simulink model "MicroMouseTemplate"  (R2024b)
settings: Solver=FixedStepAuto  StartTime=0.0  StopTime=10.0  RelTol=1e-3  EnableMultiTasking=on
undefined symbols (not defined in the file): samplingTime
settings Model: STM32="{\"DigitalPortRead\":[{\"ID\":\"MicroMouseTemplate:2483:4\"},{\"ID\":\"MicroMouseTemplate:2483:3\"}],\"DigitalPortWrite\":[{\"ID\":\"MicroMouseTemplate:84:10\"},{\"ID\":\"MicroMouseTemplate:84:9\"},{\"ID\":\"MicroMouseTemplate:84:8\"},{\"ID\":\"MicroMouseTemplate:84:7\"},{\"ID\":\"MicroMouseTemplate:84:6\"},{\"ID\":\"MicroMouseTemplate:84:5\"},{\"ID\":\"MicroMouseTemplate:84:4\"},{\"ID\":\"MicroMouseTemplate:84:3\"},{\"ID\":\"MicroMouseTemplate:2479:8\"},{\"ID\":\"MicroMouseTemplate:2479:7\"},{\"ID\":\"MicroMouseTemplate:2479:6\"},{\"ID\":\"MicroMouseTemplate:2479:4\"},{\"ID\":\"MicroMouseTemplate:160:19\"}],\"PWMOutput\":[{\"ID\":\"MicroMouseTemplate:160:25\"},{\"ID\":\"MicroMouseTemplate:160:24\"}],\"AnalogInput\":{\"ID\":\"MicroMouseTemplate:2357:1\"}}"  SimulationMode=external  ExtModeTrigDuration=10  Creator=JesseJabezArendse  LastModifiedBy=emanu
settings SolverCC: AllowMultiTaskInputOutput=on  AutoInsertRateTranBlk=on  InsertRTBMode=Never (minimum delay)
settings OptimizationCC: EnhancedBackFolding=on  PassReuseOutputArgsAs=Individual arguments  StateBitsets=on  DataBitsets=on  ZeroExternalMemoryAtStartup=off  ZeroInternalMemoryAtStartup=off  NoFixptDivByZeroProtection=on  MaxStackSize=512  OptimizeBlockOrder=speed  DifferentSizesBufferReuse=on  EfficientTunableParamExpr=on
settings DebuggingCC: MultiTaskCondExecSysMsg=none  ParameterOverflowMsg=none  ParameterPrecisionLossMsg=none  ParameterTunabilityLossMsg=error
settings HardwareCC: ProdBitPerPointer=32  ProdBitPerSizeT=32  ProdBitPerPtrDiffT=32  ProdLargestAtomicInteger=Long  ProdLargestAtomicFloat=Double  ProdWordSize=32  ProdLongLongMode=on  ProdHWDeviceType=ARM Compatible->ARM Cortex  TargetBitPerPointer=64  TargetBitPerSizeT=64  TargetBitPerPtrDiffT=64  TargetLongLongMode=on  TargetIntDivRoundTo=Zero  TargetEndianess=LittleEndian  TargetWordSize=64  TargetHWDeviceType=MATLAB Host
settings ModelReferenceCC: EnableParallelModelReferenceBuilds=on  ParallelModelReferenceMATLABWorkerInit=Copy Base Workspace  SupportModelReferenceSimTargetCustomCode=on
settings SFSimCC: MATLABDynamicMemAlloc=off  SimHardwareAcceleration=native
settings RTWCC: Description=Embedded Coder  SystemTargetFile=ert.tlc  HardwareBoard=STM32L4xx Based  TLCOptions=-p0 -aInlineSetEventsForThisBaseRateFcn=TLC_FALSE -aSuppressMultiTaskScheduler=TLC_FALSE -aRateBasedStepFcn=1  TemplateMakefile=ert_default_tmf  Toolchain=GNU Tools for ARM Embedded Processors  CodeExecutionProfiling=on  CodeProfilingInstrumentation=coarse  GPUComputeCapability=3.5
settings RTWCC: CustomHeaderCode=|
  | #include "MicroMouseProgramming\Core\Inc\IMU.h"
  | #include "MicroMouseProgramming\Core\Inc\CustomWhile.h"
  | #include "MicroMouseProgramming\Core\Inc\Motors.h"
settings RTWCC: CustomInclude=|
  | MicroMouseProgramming\Core\Inc\
  | MicroMouseProgramming\Core\Src\
settings RTWCC: CustomSource=|
  | MicroMouseProgramming\Core\Src\IMU.c
  | MicroMouseProgramming\Core\Src\CustomWhile.c
  | MicroMouseProgramming\Core\Src\Motors.c
settings CodeAppCC: ForceParamTrailComments=on  IgnoreCustomStorageClasses=off  OperatorAnnotations=on  SimulinkDataObjDesc=on  SFDataObjDesc=on  InsertBlockDesc=on
settings ERTTargetCC: CodeReplacementLibrary=ARM Cortex-M  SupportNonFinite=off  SupportComplex=off  ExtModeTransport=3  ExtModeStaticAlloc=on  ExtModeStaticAllocSize=2048  ExtModeMexFile=ext_xcp  ExtModeIntrfLevel=Level2 - Open  InlinedParameterPlacement=Hierarchical  DynamicArrayContainerType=coder::array

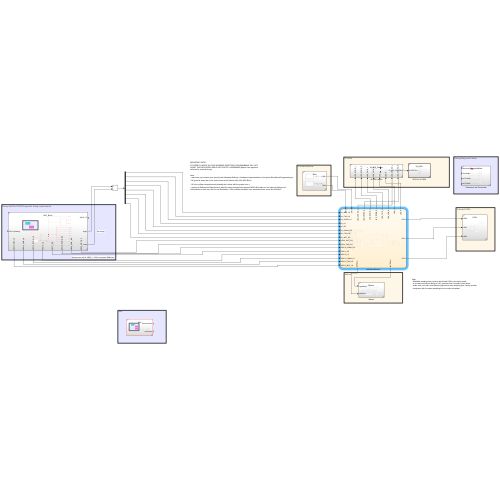
[thumbnail: Simulink's stored preview of the top-level diagram]
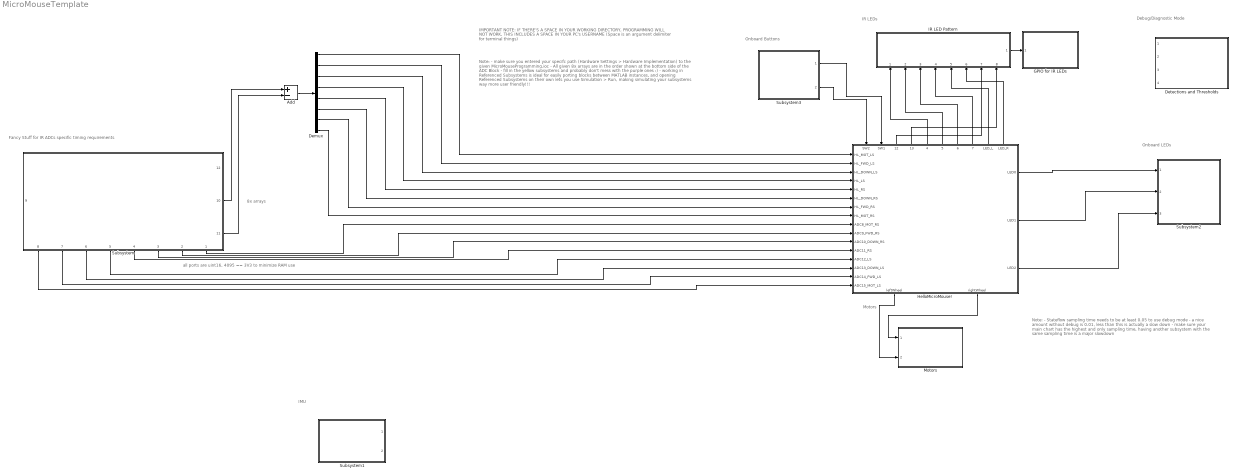
== system MicroMouseTemplate ==
  note: IMPORTANT NOTE:
      | IF THERE'S A SPACE IN YOUR WORKING DIRECTORY, PROGRAMMING WILL NOT WORK, THIS INCLUDES A SPACE IN YOUR PC's USERNAME (Space is an argument delimiter for terminal things)
  note: Note:
      | - make sure you entered your specifc path (Hardware Settings > Hardware Implementation) to the given MicroMouseProgramming.ioc
      | - All given 8x arrays are in the order shown at the bottom side of the ADC Block
      |
      | - fill in the yellow subsystems and probably don't mess with the purple ones :)
      | - working in Referenced Subsystems is ideal for easily porting blocks between MATLAB instances, and opening Referenced Subsystems on their own lets you use Simulation > Run, making simulating your subsystems way more user friendly!!!
  note: 8x arrays
  note: all ports are uint16, 4095 == 3V3 to minimize RAM use
  note: IMU
  note: Note:
      | - Stateflow sampling time needs to be at least 0.05 to use debug mode
      | - a nice amount without debug is 0.01, less than this is actually a slow down
      | - make sure your main chart has the highest and only sampling time, having another
      | subsystem with the same sampling time is a major slowdown
  note: Fancy Stuff for IR ADCs specific timing requirements
  note: IR LEDs
  note: Motors
  note: Onboard Buttons
  note: Onboard LEDs
  note: Debug/Diagnostic Mode
  Add : Sum  Inputs=+-
  Demux : Demux  Outputs=8
  Detections and Thresholds : Subsystem  ReferencedSubsystem=DiagnosticMode
  GPIO for IR LEDs : Subsystem  TreatAsAtomicUnit=on  SystemSampleTime=samplingTime  ReferencedSubsystem=IR_LEDs
  HelloMicroMouse! : Stateflow chart  TreatAsAtomicUnit=on
      settings: PortSchema="{\"entries\":[{\"content\":{\"sides\":[{\"content\":{\"connectorIds\":[\"In1\",\"In2\",\"In3\",\"In4\",\"In5\",\"In6\",\"In7\",\"In8\",\"In9\",\"In14\",\"In18\",\"In13\",\"In12\",\"In17\",\"In11\",\"In10\"]},\"type\":\"ConnectorPlacement.EquallySpacedRectSide\",\"uuid\":\"f52daa4f-6374-42e5-9ef1-0ccc99d09b58\"},{\"content\":{\"connectorIds\":[\"Out1\",\"Out10\",\"Out11\"],\"side\":\"RIGHT\"},\"type\":\"ConnectorPlacement.EquallySpacedRectSide\",\"uuid\":\"94b478cc-4dde-45c7-a588-77cf2b43cdb7\"},{\"content\":{\"connectorIds\":[\"In15\",\"In16\",\"Out12\",\"Out13\",\"Out4\",\"Out5\",\"Out6\",\"Out7\",\"Out8\",\"Out9\"],\"side\":\"TOP\"},\"type\":\"ConnectorPlacement.EquallySpacedRectSide\",\"uuid\":\"afff2079-ea5c-423e-9722-09c3bbce433b\"},{\"content\":{\"connectorIds\":[\"Out2\",\"Out3\"],\"side\":\"BOTTOM\"},\"type\":\"ConnectorPlacement.EquallySpacedRectSide\",\"uuid\":\"94e93a1d-795d-41a3-b2d8-d520b2bf47ef\"}]},\"type\":\"ConnectorPlacement.EquallySpacedConnector\",\"uuid\":\"d4d35636-54af-48ac-af70-d56caef5e090\"}],\"packageUris\":[\"http://schema.mathworks.com/mf0/Connector/R2020b\"],\"version\":\"1.0\"}"
  IR LED Pattern : Subsystem  ReferencedSubsystem=IR_LED_Pattern
      settings: PortSchema="{\"entries\":[{\"content\":{\"sides\":[{\"content\":{},\"type\":\"ConnectorPlacement.EquallySpacedRectSide\",\"uuid\":\"bebb72a7-933c-42e2-8276-ac4f31a32b24\"},{\"content\":{\"connectorIds\":[\"Out1\"],\"side\":\"RIGHT\"},\"type\":\"ConnectorPlacement.EquallySpacedRectSide\",\"uuid\":\"e4b34d82-914a-4887-8037-8bf6431a0d23\"},{\"content\":{\"side\":\"TOP\"},\"type\":\"ConnectorPlacement.EquallySpacedRectSide\",\"uuid\":\"ed031d14-68a8-4388-b5b1-46c816d5e9fd\"},{\"content\":{\"connectorIds\":[\"In1\",\"In2\",\"In3\",\"In4\",\"In5\",\"In6\",\"In7\",\"In8\"],\"side\":\"BOTTOM\"},\"type\":\"ConnectorPlacement.EquallySpacedRectSide\",\"uuid\":\"6e67ad9a-4e98-4619-ae48-9c2fca2dcbe5\"}]},\"type\":\"ConnectorPlacement.EquallySpacedConnector\",\"uuid\":\"adfb9536-7ba5-4314-9198-973b8beb12df\"}],\"packageUris\":[\"http://schema.mathworks.com/mf0/Connector/R2020b\"],\"version\":\"1.0\"}"
  Motors : Subsystem  ReferencedSubsystem=Motors
  Subsystem : Subsystem  ReferencedSubsystem=ADC_Block
      settings: PortSchema="{\"entries\":[{\"content\":{\"sides\":[{\"content\":{},\"type\":\"ConnectorPlacement.EquallySpacedRectSide\",\"uuid\":\"be6b81d5-7a49-4e34-b35f-0c07892094fc\"},{\"content\":{\"connectorIds\":[\"Out1\",\"Out2\",\"Out3\",\"Out4\",\"Out5\",\"Out6\",\"Out7\",\"Out8\"],\"side\":\"RIGHT\"},\"type\":\"ConnectorPlacement.EquallySpacedRectSide\",\"uuid\":\"5e22590a-b7c0-4c63-8de4-8d81fd6c3849\"},{\"content\":{\"connectorIds\":[\"Out12\",\"Out10\",\"Out11\"],\"side\":\"TOP\"},\"type\":\"ConnectorPlacement.EquallySpacedRectSide\",\"uuid\":\"da97636e-cea0-4a10-8fe5-d807f9ee999f\"},{\"content\":{\"connectorIds\":[\"Out9\"],\"side\":\"BOTTOM\"},\"type\":\"ConnectorPlacement.EquallySpacedRectSide\",\"uuid\":\"a593d780-81a8-4730-a8bc-2bbf356cafe4\"}]},\"type\":\"ConnectorPlacement.EquallySpacedConnector\",\"uuid\":\"0bcac921-e51a-4437-9183-315712d0a8c2\"}],\"packageUris\":[\"http://schema.mathworks.com/mf0/Connector/R2020b\"],\"version\":\"1.0\"}"
  Subsystem1 : Subsystem  ReferencedSubsystem=IMU
  Subsystem2 : Subsystem  ReferencedSubsystem=LEDs
  Subsystem3 : Subsystem  ReferencedSubsystem=SWs
  wires:
  Subsystem3/1 -> HelloMicroMouse!/16(SW1)
  Subsystem3/2 -> HelloMicroMouse!/15(SW2)
  HelloMicroMouse!/1(LED0) -> Subsystem2/1
  HelloMicroMouse!/3(rightWheel) -> Motors/1
  IR LED Pattern/1 -> GPIO for IR LEDs/1
  HelloMicroMouse!/4(LED_DOWN_L) -> IR LED Pattern/1
  HelloMicroMouse!/5(LED_DOWN_R) -> IR LED Pattern/2
  HelloMicroMouse!/2(leftWheel) -> Motors/2
  HelloMicroMouse!/6(LED_FWD_L) -> IR LED Pattern/3
  HelloMicroMouse!/7(LED_FWD_R) -> IR LED Pattern/4
  HelloMicroMouse!/8(LED_L) -> IR LED Pattern/5
  HelloMicroMouse!/9(LED_R) -> IR LED Pattern/6
  Subsystem/2 -> HelloMicroMouse!/14(ADC9_FWD_RS)
  Subsystem/3 -> HelloMicroMouse!/18(ADC10_DOWN_RS)
  Subsystem/4 -> HelloMicroMouse!/13(ADC11_RS)
  Subsystem/5 -> HelloMicroMouse!/12(ADC12_LS)
  Subsystem/6 -> HelloMicroMouse!/17(ADC13_DOWN_LS)
  Subsystem/7 -> HelloMicroMouse!/11(ADC14_FWD_LS)
  HelloMicroMouse!/10(LED1) -> Subsystem2/2
  HelloMicroMouse!/11(LED2) -> Subsystem2/3
  Subsystem/8 -> HelloMicroMouse!/10(ADC15_MOT_LS)
  Subsystem/1 -> HelloMicroMouse!/9(ADC8_MOT_RS)
  HelloMicroMouse!/12(LED_CROSS_L) -> IR LED Pattern/7
  HelloMicroMouse!/13(LED_CROSS_R) -> IR LED Pattern/8
  Subsystem/10 -> Add/1
  Subsystem/11 -> Add/2
  Add/1 -> Demux/1
  Demux/1 -> HelloMicroMouse!/1(HL_MOT_LS)
  Demux/2 -> HelloMicroMouse!/2(HL_FWD_LS)
  Demux/3 -> HelloMicroMouse!/3(HL_DOWN_LS)
  Demux/4 -> HelloMicroMouse!/4(HL_LS)
  Demux/5 -> HelloMicroMouse!/5(HL_RS)
  Demux/6 -> HelloMicroMouse!/6(HL_DOWN_RS)
  Demux/7 -> HelloMicroMouse!/7(HL_FWD_RS)
  Demux/8 -> HelloMicroMouse!/8(HL_MOT_RS)

== stateflow chart MicroMouseTemplate/HelloMicroMouse! ==
  state WallCalibrationSequence
    entry:
    LED0 = false;
    %IR LEDs
    LED_DOWN_L = 1;
    LED_DOWN_R = 1;
    LED_FWD_L = 1;
    LED_FWD_R = 1;
    LED_L = 1;
    LED_R = 1;
    LED_CROSS_L = 1;
    LED_CROSS_R = 1;
    %No Wall Readings
    LNoWall1 = 0;
    LNoWall2 = 0;
    LNoWall3 = 0;
    LNoWallAvg = 0;
    RNoWall1 = 0;
    RNoWall2 = 0;
    RNoWall3 = 0;
    RNoWallAvg = 0;
    %Wall Readings
    LWall1 = 0;
    LWall2 = 0;
    LWall3 = 0;
    LWallAvg = 0;
    RWall1 = 0;
    RWall2 = 0;
    RWall3 = 0;
    RWallAvg = 0;
    %Thresholds
    FWD_L_UPPER = 0;
    FWD_L_LOWER = 0;
    FWD_R_UPPER = 0;
    FWD_R_LOWER = 0;
    state WaitForIRLEDs
    state NoWall
      entry:
      LED0=true;
      state Reading1
        entry:
        LNoWall1=ADC14_FWD_LS;
        RNoWall1=ADC9_FWD_RS;
      state Turn
        entry:
        leftWheel=75;
        rightWheel=-75;
      state Reading2
        entry:
        leftWheel=0;
        rightWheel=0;
        LNoWall2=ADC14_FWD_LS;
        RNoWall2=ADC9_FWD_RS;
      state Turn
        entry:
        leftWheel=75;
        rightWheel=-75;
      state Reading3
        entry:
        leftWheel=0;
        rightWheel=0;
        LNoWall3=ADC14_FWD_LS;
        RNoWall3=ADC9_FWD_RS;
      state Average
        entry:
        LNoWallAvg=(1/3)*(LNoWall1+LNoWall2+LNoWall3);
        RNoWallAvg=(1/3)*(RNoWall1+RNoWall2+RNoWall3);
        LED0 = false;
      (default) -> WallCalibrationSequence.NoWall.Reading1
      WallCalibrationSequence.NoWall.Reading1 -> WallCalibrationSequence.NoWall.Turn : after(0.5,sec)
      WallCalibrationSequence.NoWall.Turn -> WallCalibrationSequence.NoWall.Reading2 : after(1,sec)
      WallCalibrationSequence.NoWall.Reading2 -> WallCalibrationSequence.NoWall.Turn : after(0.5,sec)
      WallCalibrationSequence.NoWall.Turn -> WallCalibrationSequence.NoWall.Reading3 : after(1,sec)
      WallCalibrationSequence.NoWall.Reading3 -> WallCalibrationSequence.NoWall.Average : after(0.5,sec)
    state Wall
      entry:
      LED1=true;
      state Reading1
        entry:
        LWall1=ADC14_FWD_LS;
        RWall1=ADC9_FWD_RS;
      state Turn1
        entry:
        leftWheel=75;
        rightWheel=-75;
      state Reading2
        entry:
        leftWheel=0;
        rightWheel=0;
        LWall2=ADC14_FWD_LS;
        RWall2=ADC9_FWD_RS;
      state Turn
        entry:
        leftWheel=75;
        rightWheel=-75;
      state Reading3
        entry:
        leftWheel=0;
        rightWheel=0;
        LWall3=ADC14_FWD_LS;
        RWall3=ADC9_FWD_RS;
      state Average
        entry:
        LWallAvg=(1/3)*(LWall1+LWall2+LWall3);
        RWallAvg=(1/3)*(RWall1+RWall2+RWall3);
        LED1 = false;
      (default) -> WallCalibrationSequence.Wall.Reading1
      WallCalibrationSequence.Wall.Reading1 -> Turn1 : after(0.5,sec)
      Turn1 -> WallCalibrationSequence.Wall.Reading2 : after(1,sec)
      WallCalibrationSequence.Wall.Reading2 -> WallCalibrationSequence.Wall.Turn : after(0.5,sec)
      WallCalibrationSequence.Wall.Turn -> WallCalibrationSequence.Wall.Reading3 : after(1,sec)
      WallCalibrationSequence.Wall.Reading3 -> WallCalibrationSequence.Wall.Average : after(0.5,sec)
    state FwdWeightedThresholds
      entry:
      FWD_L_UPPER=(1/3)*LNoWallAvg+(2/3)*LWallAvg;
      FWD_L_LOWER=(2/3)*LNoWallAvg+(1/3)*LWallAvg;
      FWD_R_UPPER=(1/3)*RNoWallAvg+(2/3)*RWallAvg;
      FWD_R_LOWER=(2/3)*RNoWallAvg+(1/3)*RWallAvg;
      end
      during:
      LED0=~LED0;
    (default) -> WallCalibrationSequence.WaitForIRLEDs
    WallCalibrationSequence.WaitForIRLEDs -> NoWall : [SW1]
    WallCalibrationSequence.Wall -> FwdWeightedThresholds : [SW1]
    NoWall -> WallCalibrationSequence.Wall : [SW1]
  state LineFollowing
    entry:
    LED0 = false;
    LED_DOWN_L = 1;
    LED_DOWN_R = 1;
    LED_FWD_L = 1;
    LED_FWD_R = 1;
    LED_L = 0;
    LED_R = 0;
    LED_CROSS_L = 0;
    LED_CROSS_R = 0;
    state Forward
      entry:
      leftWheel = -85;
      rightWheel = -85;
    state TurnRight
      entry:
      leftWheel = -75;
      rightWheel = 0;
    state TurnLeft
      entry:
      leftWheel = 0;
      rightWheel = -75;
    state Stop
      entry:
      leftWheel = 0;
      rightWheel = 0;
      state Wall
      state Flip
        entry:
        %if(HL_LS>2978)
        % leftWheel = -75;
        %rightWheel = 75;
        %end
        %if(HL_RS>3102)
        leftWheel = 75;
        rightWheel = -75;
        %end
      state Stop
        entry:
        leftWheel = 0;
        rightWheel = 0;
      (default) -> LineFollowing.Stop.Wall
      LineFollowing.Stop.Wall -> Flip : after(0.5,sec)
      Flip -> LineFollowing.Stop.Stop : after(60,sec)
    (default) -> LineFollowing.Forward
    TurnRight -> LineFollowing.Forward : [ADC10_DOWN_RS<3800]
    TurnLeft -> LineFollowing.Forward : [ADC13_DOWN_LS<3900]
    LineFollowing.Forward -> TurnRight [order 2] : [ADC10_DOWN_RS>3900]
    LineFollowing.Forward -> TurnLeft [order 1] : [ADC13_DOWN_LS>3850]
    LineFollowing.Forward -> LineFollowing.Stop [order 3] : [ADC14_FWD_LS>2800||ADC9_FWD_RS>2800]
    LineFollowing.Stop -> LineFollowing.Forward : [ADC14_FWD_LS<2200&&ADC9_FWD_RS<2500]
  state Stop
    entry:
    LED0 = false;
    LED_DOWN_L = 0;
    LED_DOWN_R = 0;
    LED_FWD_L = 0;
    LED_FWD_R = 0;
    LED_L = 0;
    LED_R = 0;
    LED_CROSS_L = 0;
    LED_CROSS_R = 0;
    leftWheel = 0;
    rightWheel = 0;
  state StandBy
    during:
    LED0 = ~LED0;
  state LineCalibrationSequence
    entry:
    LED0 = false;
    %IR LEDs
    LED_DOWN_L = 1;
    LED_DOWN_R = 1;
    LED_FWD_L = 1;
    LED_FWD_R = 1;
    LED_L = 1;
    LED_R = 1;
    LED_CROSS_L = 1;
    LED_CROSS_R = 1;
    %On the Line Readings
    LOnLine1 = 0;
    LOnLine2 = 0;
    LOnLine3 = 0;
    LOnLineAvg = 0;
    ROnLine1 = 0;
    ROnLine2 = 0;
    ROnLine3 = 0;
    ROnLineAvg = 0;
    %Off the line to the right
    ROffLineR1 = 0;
    ROffLineR2 = 0;
    ROffLineR3 = 0;
    ROffLineRAvg = 0;
    %Off the line to the left
    LOffLineL1 = 0;
    LOffLineL2 = 0;
    LOffLineL3 = 0;
    LOffLineLAvg = 0;
    %Downward thresholds
    DOWN_L_UPPER=0;
    DOWN_R_UPPER=0;
    DOWN_L_LOWER=0;
    DOWN_R_LOWER=0;
    state WaitForIRLEDs
    state OnLine
      entry:
      LED0=true;
      state Reading1
        entry:
        LOnLine1=ADC13_DOWN_LS;
        ROnLine1=ADC10_DOWN_RS;
      state MoveForward
        entry:
        leftWheel=75;
        rightWheel=75;
      state Reading2
        entry:
        leftWheel=0;
        rightWheel=0;
        LOnLine2=ADC13_DOWN_LS;
        ROnLine2=ADC10_DOWN_RS;
      state MoveForward1
        entry:
        leftWheel=75;
        rightWheel=75;
      state Reading3
        entry:
        leftWheel=0;
        rightWheel=0;
        LOnLine3=ADC13_DOWN_LS;
        ROnLine3=ADC10_DOWN_RS;
      state Average
        entry:
        LOnLineAvg=(1/3)*(LOnLine1+LOnLine2+LOnLine3);
        ROnLineAvg=(1/3)*(ROnLine1+ROnLine2+ROnLine3);
        LED0 = false;
      (default) -> LineCalibrationSequence.OnLine.Reading1
      LineCalibrationSequence.OnLine.Reading1 -> LineCalibrationSequence.OnLine.MoveForward : after(0.5,sec)
      LineCalibrationSequence.OnLine.MoveForward -> LineCalibrationSequence.OnLine.Reading2 : after(0.2,sec)
      LineCalibrationSequence.OnLine.Reading2 -> LineCalibrationSequence.OnLine.MoveForward1 : after(0.5,sec)
      LineCalibrationSequence.OnLine.MoveForward1 -> LineCalibrationSequence.OnLine.Reading3 : after(0.2,sec)
      LineCalibrationSequence.OnLine.Reading3 -> LineCalibrationSequence.OnLine.Average : after(0.5,sec)
    state OffLineR
      entry:
      LED1=true;
      state Reading1
        entry:
        ROffLineR1=ADC10_DOWN_RS;
      state MoveForward
        entry:
        leftWheel=75;
        rightWheel=75;
      state Reading2
        entry:
        leftWheel=0;
        rightWheel=0;
        ROffLineR2=ADC10_DOWN_RS;
      state MoveForward1
        entry:
        leftWheel=75;
        rightWheel=75;
      state Reading3
        entry:
        leftWheel=0;
        rightWheel=0;
        ROffLineR3=ADC10_DOWN_RS;
      state Average
        entry:
        ROffLineRAvg=(1/3)*(ROffLineR1+ROffLineR2+ROffLineR3);
        LED1 = false;
      (default) -> LineCalibrationSequence.OffLineR.Reading1
      LineCalibrationSequence.OffLineR.Reading1 -> LineCalibrationSequence.OffLineR.MoveForward : after(0.5,sec)
      LineCalibrationSequence.OffLineR.MoveForward -> LineCalibrationSequence.OffLineR.Reading2 : after(0.2,sec)
      LineCalibrationSequence.OffLineR.Reading2 -> LineCalibrationSequence.OffLineR.MoveForward1 : after(0.5,sec)
      LineCalibrationSequence.OffLineR.MoveForward1 -> LineCalibrationSequence.OffLineR.Reading3 : after(0.2,sec)
      LineCalibrationSequence.OffLineR.Reading3 -> LineCalibrationSequence.OffLineR.Average : after(0.5,sec)
    state OffLineL
      entry:
      LED2=true;
      state Reading1
        entry:
        LOffLineL1=ADC13_DOWN_LS;
      state MoveForward
        entry:
        leftWheel=75;
        rightWheel=75;
      state Reading2
        entry:
        leftWheel=0;
        rightWheel=0;
        LOffLineL2=ADC13_DOWN_LS;
      state MoveForward1
        entry:
        leftWheel=75;
        rightWheel=75;
      state Reading3
        entry:
        leftWheel=0;
        rightWheel=0;
        LOffLineL3=ADC13_DOWN_LS;
      state Average
        entry:
        LOffLineLAvg=(1/3)*(LOffLineL1+LOffLineL2+LOffLineL3);
        LED2 = false;
      (default) -> LineCalibrationSequence.OffLineL.Reading1
      LineCalibrationSequence.OffLineL.Reading1 -> LineCalibrationSequence.OffLineL.MoveForward : after(0.5,sec)
      LineCalibrationSequence.OffLineL.MoveForward -> LineCalibrationSequence.OffLineL.Reading2 : after(0.2,sec)
      LineCalibrationSequence.OffLineL.Reading2 -> LineCalibrationSequence.OffLineL.MoveForward1 : after(0.5,sec)
      LineCalibrationSequence.OffLineL.MoveForward1 -> LineCalibrationSequence.OffLineL.Reading3 : after(0.2,sec)
      LineCalibrationSequence.OffLineL.Reading3 -> LineCalibrationSequence.OffLineL.Average : after(0.5,sec)
    state DownWeightedThresholds
      entry:
      DOWN_L_UPPER=(1/3)*LOffLineLAvg+(2/3)*LOnLineAvg;
      DOWN_L_LOWER=(2/3)*LOffLineLAvg+(1/3)*LOnLineAvg;
      DOWN_R_UPPER=(1/3)*ROffLineRAvg+(2/3)*ROnLineAvg;
      DOWN_R_LOWER=(2/3)*ROffLineRAvg+(1/3)*ROnLineAvg;
      end
      during:
      LED0=~LED0;
    (default) -> LineCalibrationSequence.WaitForIRLEDs
    LineCalibrationSequence.WaitForIRLEDs -> OnLine : [SW1]
    OffLineR -> OffLineL : [SW1]
    OnLine -> OffLineR : [SW1]
    OffLineL -> DownWeightedThresholds : [SW1]
  state Forward
    entry:
    LED0 = false;
    LED1 = true;
    LED2 = false;
    %Move forward
    leftWheel = 75;
    rightWheel = 75;
  state TiltLeft
    entry:
    LED0 = true;
    LED1 = false;
    LED2 = false;
    %Turn to the right
    leftWheel = 75;
    rightWheel = 0;
  state ForwardWall
    entry:
    leftWheel = 0;
    rightWheel = 0;
    state Wall
    state Spin
      entry:
      leftWheel = 75;
      rightWheel = -75;
    state Stop
      entry:
      leftWheel = 0;
      rightWheel = 0;
    (default) -> ForwardWall.Wall
    ForwardWall.Wall -> Spin : after(0.5,sec)
    Spin -> ForwardWall.Stop : after(60,sec)
  state TiltRight
    entry:
    LED0 = false;
    LED1 = false;
    LED2 = true;
    %Turn to the left
    leftWheel = 0;
    rightWheel = 75;
  (default) -> StandBy [order 1]
  LineFollowing -> Stop : [SW2]
  StandBy -> LineFollowing : [SW2]
  (default) -> Forward [order 2]
  TiltRight -> Forward [order 1] : [ADC10_DOWN_RS<2500&&ADC13_DOWN_LS>1900]
  TiltLeft -> Forward [order 1] : [ADC10_DOWN_RS>2200&&ADC13_DOWN_LS<2000]
  Forward -> TiltLeft [order 2] : [ADC10_DOWN_RS<1900&&ADC13_DOWN_LS>2400]
  Forward -> TiltRight [order 1] : [ADC10_DOWN_RS>3000&&ADC13_DOWN_LS<1500]
  Forward -> ForwardWall [order 3] : [ADC14_FWD_LS>2200||ADC9_FWD_RS>3500]
  ForwardWall -> Forward : [ADC14_FWD_LS<1700&&ADC9_FWD_RS<3100]
  TiltLeft -> ForwardWall [order 2] : [ADC14_FWD_LS>2200||ADC9_FWD_RS>3500]
  TiltRight -> ForwardWall [order 2] : [ADC14_FWD_LS>2200||ADC9_FWD_RS>3500]
  data: HL_MOT_LS input; HL_FWD_LS input; HL_DOWN_LS input; HL_LS input; HL_RS input; HL_DOWN_RS input; HL_FWD_RS input; HL_MOT_RS input; ADC8_MOT_RS input; ADC15_MOT_LS input; ADC14_FWD_LS input; ADC12_LS input; ADC11_RS input; ADC9_FWD_RS input; SW2 input; LED0 output; SW1 input; leftWheel output int16; rightWheel output int16; LED_DOWN_L output; LED_DOWN_R output; ADC13_DOWN_LS input; ADC10_DOWN_RS input; LED_FWD_L output; LED_FWD_R output; LED_L output; LED_R output; LED1 output; LED2 output; LED_CROSS_L output; LED_CROSS_R output; FWD_L_UPPER local; FWD_R_LOWER local; LNoWall1 local; RNoWall3 local; LNoWall2 local; LNoWall3 local; LNoWallAvg local; LWall1 local; LWall2 local; LWall3 local; LWallAvg local; RNoWall1 local; RNoWall2 local; RNoWallAvg local; RWall1 local; RWall2 local; RWall3 local; RWallAvg local; FWD_R_UPPER local; FWD_L_LOWER local; LOffLineL1 local; LOffLineL2 local; LOffLineL3 local; LOffLineLAvg local; LOffLineR1 local; LOffLineR2 local; LOffLineR3 local; LOffLineRAvg local; LOnLine1 local; LOnLine2 local; LOnLine3 local; LOnLineAvg local; ROffLineL1 local; ROffLineL2 local; ROffLineL3 local; ROffLineLAvg local; ROffLineR1 local; ROffLineR2 local; ROffLineR3 local; ROffLineRAvg local; ROnLine1 local; ROnLine2 local; ROnLine3 local; ROnLineAvg local; DOWN_L_LOWER local; DOWN_L_UPPER local; DOWN_R_LOWER local; DOWN_R_UPPER local
